simulink model "hw3_3_e_sim"  (R2024a)
settings: Solver=VariableStepAuto  StartTime=0.0  StopTime=30  RelTol=1e-3
values from neighbouring files (symbols this model uses):
  A_est = Gd_ss.A - L*Gd_ss.C    [hw3_3_e.m]
  B_est = [Gd_ss.B L]    [hw3_3_e.m]
  Gd_ss = ss(Gd_tf)    [hw3_3_a.m]    (also in hw3_3_b.m; hw3_3_c.m; hw3_3_d.m; hw3_3_e.m)
  K = place(Gd_ss.A, Gd_ss.B, p)    [hw3_3_b.m]    (also in hw3_3_c.m; hw3_3_e.m; hw3_3_f.m)
  T = 0.2    [hw3_1_a.m]    (also in hw3_1_b.m; hw3_1_c.m; hw3_1_d.m; hw3_2_a.m)
  X0 = [1; 1]    [hw3_3_c.m]    (also in hw3_3_e.m)
settings Model: Creator=vv  LastModifiedBy=vv

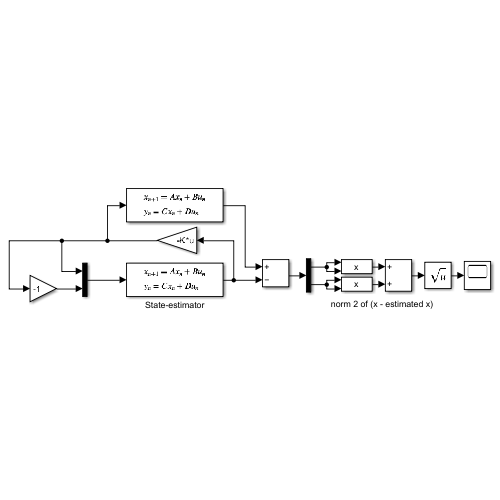
[thumbnail: Simulink's stored preview of the top-level diagram]
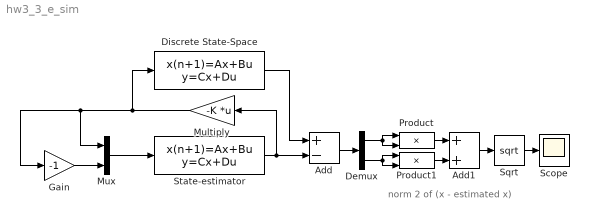
== system hw3_3_e_sim ==
  note: norm 2 of (x - estimated x)
  Add : Sum  Inputs=+-
  Add1 : Sum
  Demux : Demux  Outputs=2
  Discrete State-Space : DiscreteStateSpace  A=Gd_ss.A  B=Gd_ss.B  C=[1 0;0 1]  D=[0 ; 0]  InitialCondition=X0  SampleTime=T
  Gain : Gain  Gain=-1
  Multiply : Gain  Gain=-K  Multiplication=Matrix(K*u)
  Mux : Mux  Inputs=2
  Product : Product
  Product1 : Product
  Scope : Scope
  Sqrt : Sqrt
  State-estimator : DiscreteStateSpace  A=A_est  B=B_est  C=eye(2)  D=zeros(2,2)  SampleTime=T
  wires:
  Discrete State-Space/1 -> Add/1
  Multiply/1 -> Gain/1, Mux/1, Discrete State-Space/1
  State-estimator/1 -> Multiply/1, Add/2
  Mux/1 -> State-estimator/1
  Gain/1 -> Mux/2
  Add/1 -> Demux/1
  Demux/2 -> Product1/1, Product1/2
  Demux/1 -> Product/1, Product/2
  Product1/1 -> Add1/2
  Product/1 -> Add1/1
  Add1/1 -> Sqrt/1
  Sqrt/1 -> Scope/1
